simulink library "csu_taf_thruster_arm_fire_mtv_lib"  (R2014b)
settings: Solver=ode45  StartTime=0.0  StopTime=10.0  RelTol=1e-3
undefined symbols (not defined in the file or in its folder): taf_coarse_armed, taf_coarse_disarmed
libraries: simulink x1, util_info_lib x1
settings Model: Creator=escrane  LastModifiedBy=mstewart

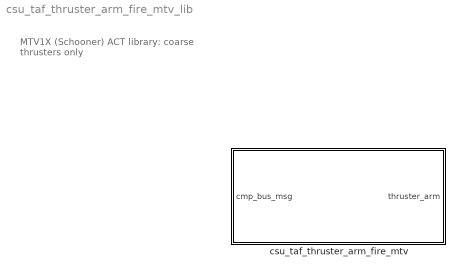
== system csu_taf_thruster_arm_fire_mtv_lib ==
  note: MTV1X (Schooner) ACT library:
      | coarse thrusters only
  csu_taf_thruster_arm_fire_mtv : Subsystem

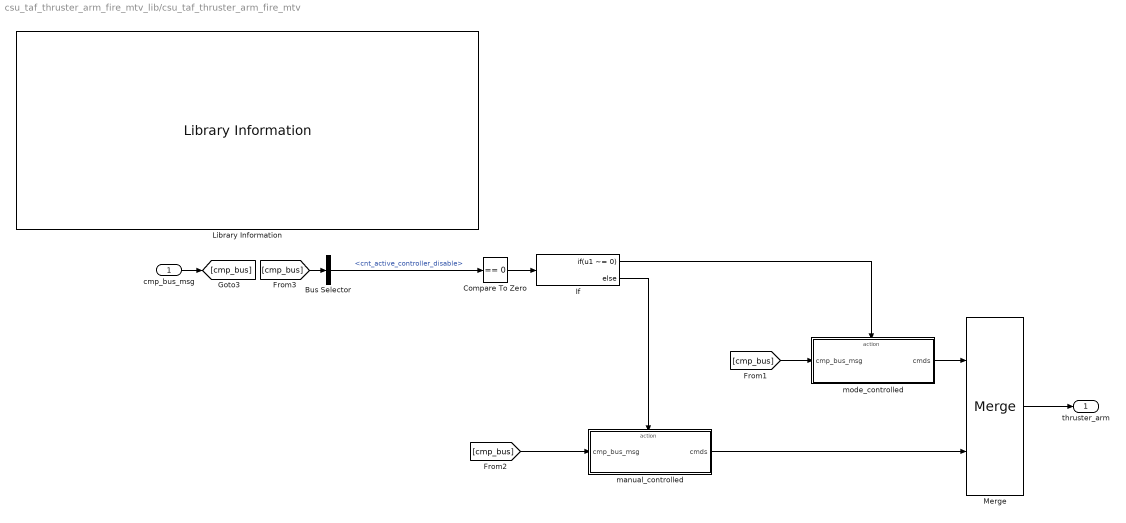
== system csu_taf_thruster_arm_fire_mtv_lib/csu_taf_thruster_arm_fire_mtv ==
  cmp_bus_msg : Inport
  Bus Selector : BusSelector  OutputSignals=cnt_active_controller_disable
  Compare To Zero : simulink/Logic and Bit Operations/Compare To Zero  relop===  OutDataTypeStr=boolean
  If : If  IfExpression=u1 ~= 0
  Library Information : util_info_lib/Library Information  owner='escrane'
  Merge : Merge
  manual_controlled : Subsystem  TreatAsAtomicUnit=on
  mode_controlled : Subsystem  TreatAsAtomicUnit=on
  thruster_arm : Outport
  wires:
  Bus Selector/1 -> Compare To Zero/1  "<cnt_active_controller_disable>"
  mode_controlled/1(cmds) -> Merge/1
  manual_controlled/1(cmds) -> Merge/2
  Merge/1 -> thruster_arm/1
  cmp_bus_msg/1 -> [cmp_bus]
  [cmp_bus] -> Bus Selector/1
  [cmp_bus] -> mode_controlled/1(cmp_bus_msg)
  Compare To Zero/1 -> If/1
  If/1 -> mode_controlled/Action
  If/2 -> manual_controlled/Action
  [cmp_bus] -> manual_controlled/1(cmp_bus_msg)

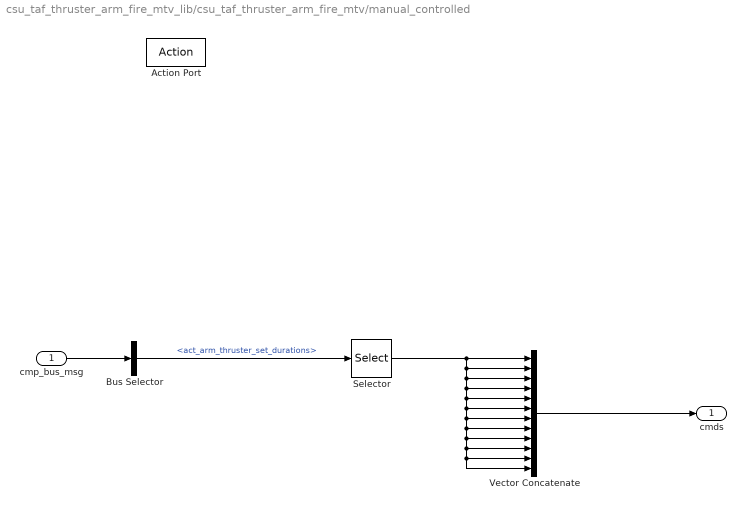
== system csu_taf_thruster_arm_fire_mtv_lib/csu_taf_thruster_arm_fire_mtv/manual_controlled ==
  cmp_bus_msg : Inport
  Action Port : ActionPort
  Bus Selector : BusSelector  OutputSignals=act_arm_thruster_set_durations
  Selector : Selector  InputPortWidth=4
  Vector Concatenate : Concatenate  NumInputs=12
  cmds : Outport
  wires:
  Vector Concatenate/1 -> cmds/1
  cmp_bus_msg/1 -> Bus Selector/1
  Selector/1 -> Vector Concatenate/2, Vector Concatenate/3, Vector Concatenate/4, Vector Concatenate/5, Vector Concatenate/6, Vector Concatenate/7, Vector Concatenate/8, Vector Concatenate/9, Vector Concatenate/10, Vector Concatenate/11, Vector Concatenate/12, Vector Concatenate/1
  Bus Selector/1 -> Selector/1  "<act_arm_thruster_set_durations>"

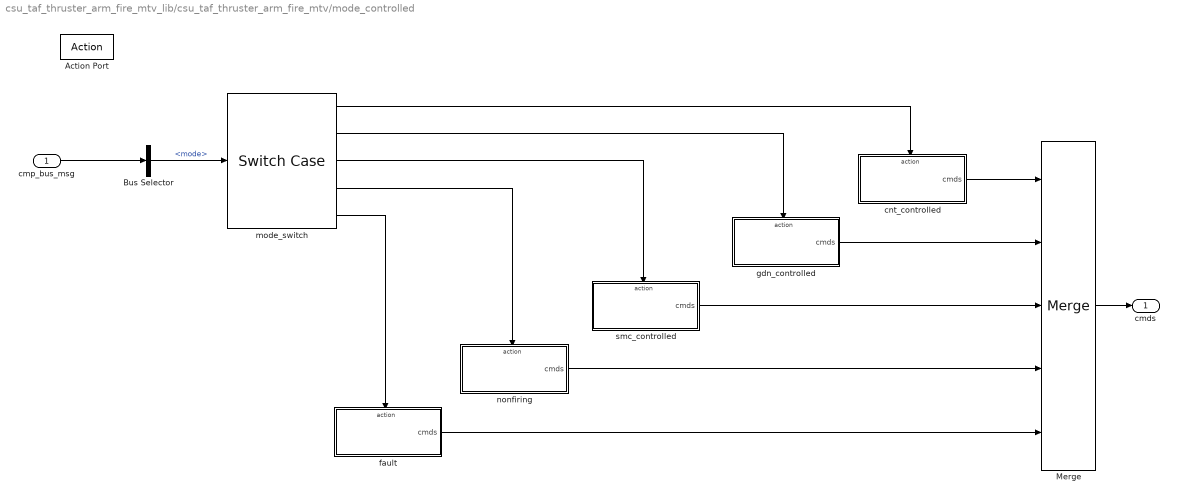
== system csu_taf_thruster_arm_fire_mtv_lib/csu_taf_thruster_arm_fire_mtv/mode_controlled ==
  cmp_bus_msg : Inport
  Action Port : ActionPort
  Bus Selector : BusSelector  OutputSignals=mode
  Merge : Merge  Inputs=5
  cnt_controlled : Subsystem  TreatAsAtomicUnit=on
  fault : Subsystem  TreatAsAtomicUnit=on
  gdn_controlled : Subsystem  TreatAsAtomicUnit=on
  mode_switch : SwitchCase  CaseConditions={ uint8(enum_mode.pointing), [uint8(enum_mode.deltav), uint8(enum_mode.deorbit), uint8(enum_mode.braking) uint8(enum_mode.landing)], uint8(enum_mode.safe), [uint8(enum_mode.startup), uint8(enum_mode.surface), uint8(enum_mode.safesurface)]}
  nonfiring : Subsystem  TreatAsAtomicUnit=on
  smc_controlled : Subsystem  TreatAsAtomicUnit=on
  cmds : Outport
  wires:
  cnt_controlled/1(cmds) -> Merge/1
  mode_switch/1 -> cnt_controlled/Action
  Bus Selector/1 -> mode_switch/1  "<mode>"
  mode_switch/2 -> gdn_controlled/Action
  mode_switch/3 -> smc_controlled/Action
  mode_switch/4 -> nonfiring/Action
  gdn_controlled/1(cmds) -> Merge/2
  smc_controlled/1(cmds) -> Merge/3
  nonfiring/1(cmds) -> Merge/4
  Merge/1 -> cmds/1
  mode_switch/5 -> fault/Action
  fault/1(cmds) -> Merge/5
  cmp_bus_msg/1 -> Bus Selector/1

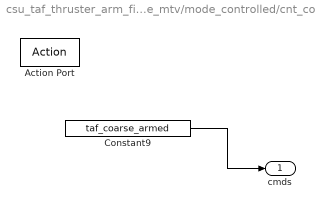
== system csu_taf_thruster_arm_fire_mtv_lib/csu_taf_thruster_arm_fire_mtv/mode_controlled/cnt_controlled ==
  Action Port : ActionPort
  Constant9 : Constant  Value=taf_coarse_armed  OutDataTypeStr=uint32
  cmds : Outport
  wires:
  Constant9/1 -> cmds/1

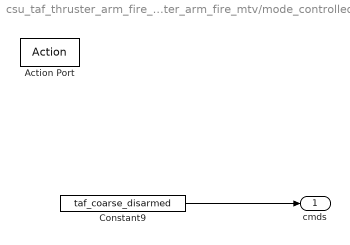
== system csu_taf_thruster_arm_fire_mtv_lib/csu_taf_thruster_arm_fire_mtv/mode_controlled/fault ==
  Action Port : ActionPort
  Constant9 : Constant  Value=taf_coarse_disarmed  OutDataTypeStr=uint32
  cmds : Outport
  wires:
  Constant9/1 -> cmds/1

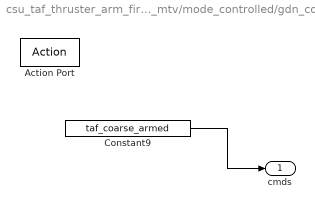
== system csu_taf_thruster_arm_fire_mtv_lib/csu_taf_thruster_arm_fire_mtv/mode_controlled/gdn_controlled ==
  Action Port : ActionPort
  Constant9 : Constant  Value=taf_coarse_armed  OutDataTypeStr=uint32
  cmds : Outport
  wires:
  Constant9/1 -> cmds/1

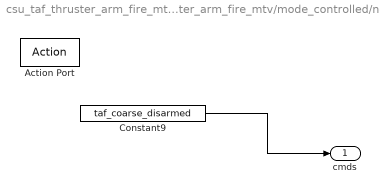
== system csu_taf_thruster_arm_fire_mtv_lib/csu_taf_thruster_arm_fire_mtv/mode_controlled/nonfiring ==
  Action Port : ActionPort
  Constant9 : Constant  Value=taf_coarse_disarmed  OutDataTypeStr=uint32
  cmds : Outport
  wires:
  Constant9/1 -> cmds/1

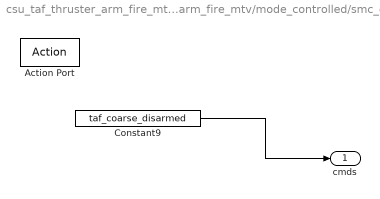
== system csu_taf_thruster_arm_fire_mtv_lib/csu_taf_thruster_arm_fire_mtv/mode_controlled/smc_controlled ==
  Action Port : ActionPort
  Constant9 : Constant  Value=taf_coarse_disarmed  OutDataTypeStr=uint32
  cmds : Outport
  wires:
  Constant9/1 -> cmds/1
